simulink model "FOC_CURRENTLOOP_DOUBLE"  (R2024a)
settings: Solver=FixedStepDiscrete  StartTime=0.0  StopTime=10.0  FixedStep=TsBSP  RelTol=1e-3
values from neighbouring files (symbols this model uses):
  bandwidth = 1256.6370614359173    [FOC_CURRENTLOOP_DOUBLE.sldd]
  flux = 0.0109    [FOC_CURRENTLOOP_DOUBLE.sldd]
  Ls = 0.000195185    [FOC_CURRENTLOOP_DOUBLE.sldd]
  Polepairs = 5.0    [FOC_CURRENTLOOP_DOUBLE.sldd]
  Polepairs_MODEL = 5.0    [FOC_CURRENTLOOP_DOUBLE.sldd]
  PWMHalfPeriod = 4199.0    [FOC_CURRENTLOOP_DOUBLE.sldd]
  PWMHalfPeriod_MODEL = 4199.0    [FOC_CURRENTLOOP_DOUBLE.sldd]
  Rs = 0.1763    [FOC_CURRENTLOOP_DOUBLE.sldd]
  TsBSP = 5.0E-5    [FOC_CURRENTLOOP_DOUBLE.sldd]
  TsFOC = 0.0001    [FOC_CURRENTLOOP_DOUBLE.sldd]
undefined symbols (not defined in the file or in its folder): sigbuilder_block
libraries: slpidlib x2, mcbplantlib x1, SignalEditorBlockLib x1, autolibpmsmexterior x1
(part 1 of 2)
settings Model: DataDictionary=FOC_CURRENTLOOP_DOUBLE.sldd  Creator=beau_  LastModifiedBy=chaoli_wanjietian
settings SolverCC: AlgebraicLoopSolver=TrustRegion
settings OptimizationCC: DefaultParameterBehavior=Inlined  UseDivisionForNetSlopeComputation=on  GainParamInheritBuiltInType=on  UseFloatMulNetSlope=on  InlineInvariantSignals=on  PassReuseOutputArgsAs=Individual arguments  ZeroExternalMemoryAtStartup=off  ZeroInternalMemoryAtStartup=off  NoFixptDivByZeroProtection=on  EfficientFloat2IntCast=on  LifeSpan=1  OptimizeBlockOrder=speed  DifferentSizesBufferReuse=on  EfficientTunableParamExpr=on
settings DebuggingCC: ParameterTunabilityLossMsg=error  UnconnectedInputMsg=warning  UnconnectedOutputMsg=warning  UnconnectedLineMsg=warning  BusObjectLabelMismatch=error
settings HardwareCC: ProdBitPerPointer=32  ProdBitPerSizeT=32  ProdBitPerPtrDiffT=32  ProdLargestAtomicInteger=Long  ProdLargestAtomicFloat=Double  ProdWordSize=32  ProdLongLongMode=on  ProdHWDeviceType=ARM Compatible->ARM Cortex-M
settings ModelReferenceCC: EnableRefExpFcnMdlSchedulingChecks=on
settings SFSimCC: SimUserIncludeDirs=E:\Exp_G431\NUM1_CURRENTLOOP\  MATLABDynamicMemAlloc=off
settings SFSimCC: SimCustomHeaderCode=|
  | #include "jscl_transform.h"
  | #include "jscl_currentloop.h"
settings SFSimCC: SimUserSources=|
  | jscl_transform.c
  | jscl_currentloop.c
settings RTWCC: Description=Embedded Coder  SystemTargetFile=ert.tlc  GenCodeOnly=on  TemplateMakefile=ert_default_tmf  GenerateReport=on  CustomInclude=E:\Exp_G431\NUM1_CURRENTLOOP  IncludeHyperlinkInReport=on  LaunchReport=on  GenerateTraceInfo=on  GPUComputeCapability=3.5  DLArmComputeVersion=19.05
settings RTWCC: CustomHeaderCode=|
  | #include "jscl_clarke.h"
  | #include "jscl_park.h"
settings RTWCC: CustomSource=|
  | jscl_clarke.c
  | jscl_park.c
settings CodeAppCC: GenerateComments=off  IgnoreCustomStorageClasses=off  OperatorAnnotations=on  SimulinkDataObjDesc=on  SFDataObjDesc=on  CustomSymbolStrGlobalVar=rt$N$M  CustomSymbolStrType=$N$M  CustomSymbolStrFcn=$N$M$F  CustomSymbolStrFcnArg=param_$I$N$M  CustomSymbolStrBlkIO=local_$N$M  CustomSymbolStrMacro=$N$M  SimulinkBlockComments=off
settings ERTTargetCC: TargetLangStandard=C99 (ISO)  CodeReplacementLibrary=ARM Cortex-M  GenerateSampleERTMain=on  IncludeMdlTerminateFcn=off  CombineSignalStateStructs=on  SuppressErrorStatus=on  SupportNonFinite=off  SupportComplex=off  InlinedParameterPlacement=NonHierarchical  ERTCustomFileTemplate=example_file_process.tlc  EnableDataOwnership=on  ERTFilePackagingFormat=CompactWithDataFile  IndentSize=4

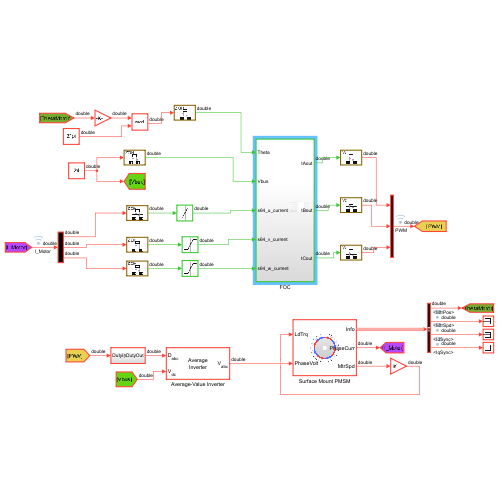
[thumbnail: Simulink's stored preview of the top-level diagram]
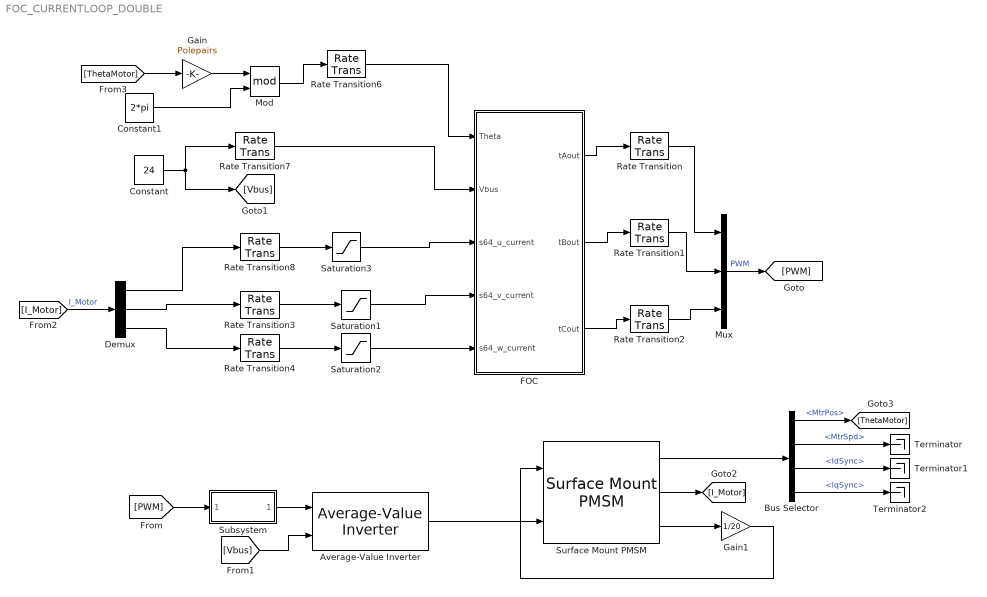
== system FOC_CURRENTLOOP_DOUBLE ==
  Average-Value Inverter : mcbplantlib/Average-Value Inverter
  Bus Selector : BusSelector  OutputSignals=MtrPos,MtrSpd,IdSync,IqSync
  Constant : Constant  Value=24  SampleTime=-1
  Constant1 : Constant  Value=2*pi  SampleTime=-1
  Demux : Demux  Outputs=3
  FOC : Subsystem
  Gain : Gain  Gain=Polepairs
  Gain1 : Gain  Gain=1/20
  Mod : Math  Operator=mod
  Mux : Mux  Inputs=3
  Rate Transition{,1..4,6..8} (8 alike) : RateTransition
  Saturation1 : Saturate  UpperLimit=50  LowerLimit=-50
  Saturation2 : Saturate  UpperLimit=50  LowerLimit=-50
  Saturation3 : Saturate  UpperLimit=50  LowerLimit=-50
  Subsystem : Subsystem
  Surface Mount PMSM : autolibpmsmexterior/Surface Mount PMSM  port_config=Torque  sim_type=Discrete  Ts=TsBSP  P=Polepairs_MODEL  Rs=Rs_MODEL  Ldq_=Ls_MODEL  KConstText=Permanent flux linkage constant (lambda_pm):  lambda_pm=flux_MODEL  Ke=159.9771  Kt=1.323  mechanical=[5.8e-4, 1.59e-4, 0]  idq0=[0 0]  theta_init=0  omega_init=0  KConst=flux_MODEL  lambda_pm_calc=flux_MODEL  RefBlkName='autolibpmsmexterior/Surface Mount PMSM'  aMode=5  Ldq="[0.0017      0.0017]"
  Terminator : Terminator
  Terminator1 : Terminator
  Terminator2 : Terminator
  wires:
  Rate Transition6/1 -> FOC/1(Theta)
  FOC/1(tAout) -> Rate Transition/1
  FOC/2(tBout) -> Rate Transition1/1
  FOC/3(tCout) -> Rate Transition2/1
  Average-Value Inverter/1 -> Surface Mount PMSM/2
  Rate Transition1/1 -> Mux/2
  Rate Transition/1 -> Mux/1
  Rate Transition2/1 -> Mux/3
  Mux/1 -> [PWM]  "PWM"
  [PWM] -> Subsystem/1(DutyIn)
  Subsystem/1(DutyOut) -> Average-Value Inverter/1
  Constant/1 -> [Vbus], Rate Transition7/1
  [Vbus] -> Average-Value Inverter/2
  Surface Mount PMSM/1 -> Bus Selector/1
  Bus Selector/1 -> [ThetaMotor]  "<MtrPos>"
  [ThetaMotor] -> Gain/1
  Gain/1 -> Mod/1
  Mod/1 -> Rate Transition6/1
  Constant1/1 -> Mod/2
  Bus Selector/2 -> Terminator/1  "<MtrSpd>"
  Bus Selector/3 -> Terminator1/1  "<IdSync>"
  Bus Selector/4 -> Terminator2/1  "<IqSync>"
  Surface Mount PMSM/3 -> Gain1/1
  Gain1/1 -> Surface Mount PMSM/1
  Rate Transition7/1 -> FOC/2(Vbus)
  Rate Transition8/1 -> Saturation3/1
  Surface Mount PMSM/2 -> [I_Motor]
  Rate Transition3/1 -> Saturation1/1
  Saturation1/1 -> FOC/4(s64_v_current)
  Saturation2/1 -> FOC/5(s64_w_current)
  Rate Transition4/1 -> Saturation2/1
  Saturation3/1 -> FOC/3(s64_u_current)
  [I_Motor] -> Demux/1  "I_Motor"
  Demux/2 -> Rate Transition3/1
  Demux/3 -> Rate Transition4/1
  Demux/1 -> Rate Transition8/1

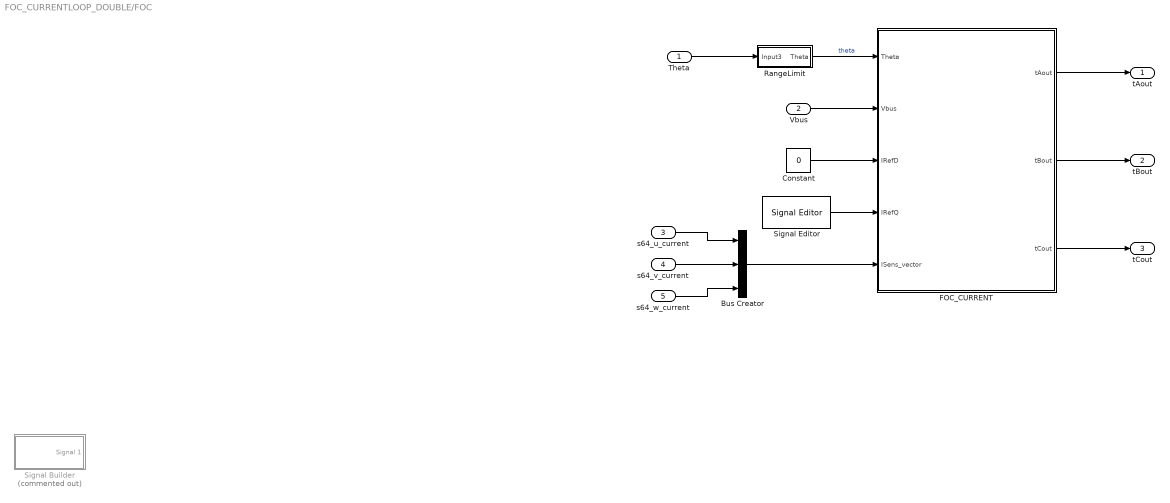
== system FOC_CURRENTLOOP_DOUBLE/FOC ==
  Theta : Inport
  Vbus : Inport  Port=2
  s64_u_current : Inport  Port=3
  s64_v_current : Inport  Port=4
  s64_w_current : Inport  Port=5
  Bus Creator : BusCreator  Inputs=3  OutDataTypeStr=Bus: VectorUVW_T
      settings: InheritFromInputs=off
  Constant : Constant  Value=0  SampleTime=-1
  FOC_CURRENT : Subsystem  TreatAsAtomicUnit=on  SystemSampleTime=TsFOC
      settings: RTWSystemCode=Nonreusable function
  RangeLimit : Subsystem
  Signal Builder : Subsystem  Tag=STV Subsys  Commented=on  LoadFcn=sigbuilder_block('load');  StartFcn=sigbuilder_block('start');  StopFcn=sigbuilder_block('stop');  ClipboardFcn=sigbuilder_block('clipboard');  mask(Sigbuilder block){tuvar=[0:10]}
      mask help: Simulink:masks:SigbuilderBlock_MD
      mask init:
      | if ~strcmp(get_param(bdroot(gcbh),'SimulationStatus'),'stopped') tuvar = sigbuilder_block('maskInit'); end
      settings: CopyFcn=sigbuilder_block('copy');  DeleteFcn=sigbuilder_block('delete');  ModelCloseFcn=sigbuilder_block('modelClose');  PreSaveFcn=sigbuilder_block('preSave');  PauseFcn=sigbuilder_block('pause');  ContinueFcn=sigbuilder_block('continue');  NameChangeFcn=sigbuilder_block('namechange');  OpenFcn=sigbuilder_block('open',[261 231.5 550.5 362.5 ]);  CloseFcn=sigbuilder_block('close');
      mask Display: plot(0, 0, 100, 100,[2, 2, 32, 32, 2], [68, 8, 8, 68, 68],[32, 2], [38, 38], [32, 19, 2],[53, 60, 44], [32, 17, 17, 2],[16, 16, 31, 31]);txt = getActiveGroup(gcbh);text(2, 100, txt,'verticalAlignment', 'top');
  Signal Editor : SignalEditorBlockLib/Signal Editor  FileName=E:\Exp_G431\NUM1_CURRENTLOOP\builder_edit.mat  ActiveScenario=Scenario  ActiveSignal=IRefQ  IsBus=off  OutputBusObjectStr=Bus: BusObject  SampleTime=TsFOC  Interpolate=off  ZeroCross=off  OutputAfterFinalValue=Setting to zero  Unit=inherit  PreserveSignalName=on  ApplySigPropsToAllScenarios=on  ApplySigPropsToAllSignals=off
  tAout : Outport
  tBout : Outport  Port=2
  tCout : Outport  Port=3
  wires:
  Vbus/1 -> FOC_CURRENT/2(Vbus)
  Theta/1 -> RangeLimit/1(Input3)
  RangeLimit/1(Theta) -> FOC_CURRENT/1(Theta)  "theta"
  Constant/1 -> FOC_CURRENT/3(IRefD)
  Signal Editor/1 -> FOC_CURRENT/4(IRefQ)
  Bus Creator/1 -> FOC_CURRENT/5(ISens_vector)
  s64_u_current/1 -> Bus Creator/1
  s64_v_current/1 -> Bus Creator/2
  s64_w_current/1 -> Bus Creator/3
  FOC_CURRENT/3(tCout) -> tCout/1
  FOC_CURRENT/2(tBout) -> tBout/1
  FOC_CURRENT/1(tAout) -> tAout/1

== system FOC_CURRENTLOOP_DOUBLE/Subsystem ==
  DutyIn : Inport
  Constant : Constant  Value=0.5
  Gain : Gain  Gain=1/PWMHalfPeriod_MODEL
  Gain1 : Gain  Gain=-1
  Sum : Sum  Inputs=|+-
  Sum1 : Sum  Inputs=|++
  DutyOut : Outport
  wires:
  DutyIn/1 -> Gain/1
  Gain/1 -> Sum/1
  Sum/1 -> Gain1/1
  Gain1/1 -> Sum1/1
  Sum1/1 -> DutyOut/1
  Constant/1 -> Sum1/2, Sum/2

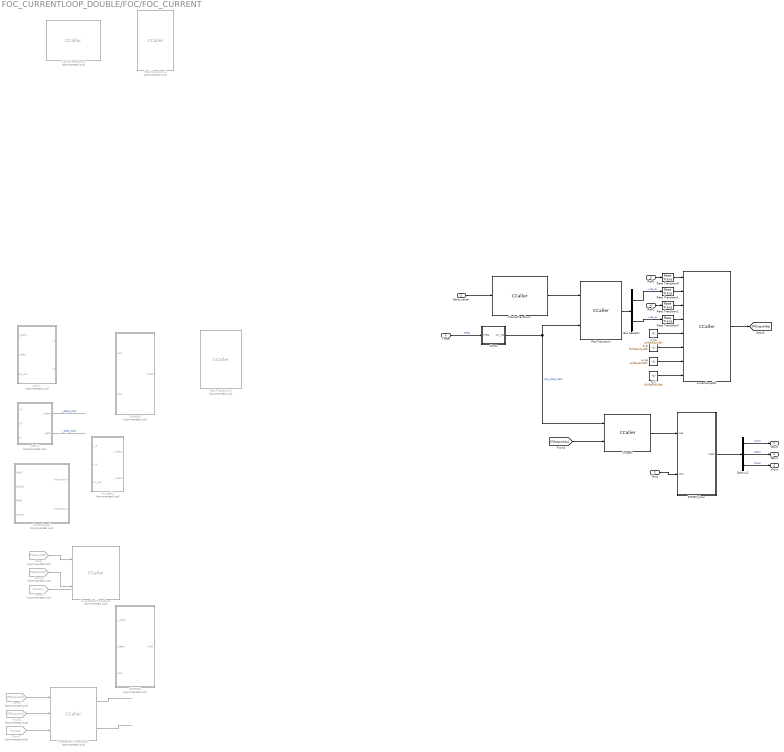
== system FOC_CURRENTLOOP_DOUBLE/FOC/FOC_CURRENT ==
  Theta : Inport
  Vbus : Inport  Port=2
  IRefD : Inport  Port=3
  IRefQ : Inport  Port=4
  ISens_vector : Inport  Port=5  OutDataTypeStr=Bus: VectorUVW_T
  Bus Selector : BusSelector  OutputSignals=s64_d,s64_q
  ClarkeTransform : CCaller  FunctionName=ClarkeTransform  PortSpecificationStruct="%)30     .    Z ,   8    (     @         %    \"     (    !     0         %  0 \"0    $    _    07)G3F%M90  4&]R=$YA;64 4V-O<&4     26YD97@     5'EP90      4VEZ90      27-';&]B86P   X    X    !@    @    $          4    (     0    8    !         !     &    04)#7VEN   .    .     8    (    !          %    \"     $    &     0         0    !@   $%\"0U]I;@  #@   #@    &    \"     0         !0    @    !    !0    $         $     4   !);G!U=     X    X    !@    @    &          4    (     0    $    !          D    (               .    0     8    (    !          %    \"     $    0     0         0    $    $)U<SH@5F5C=&]R55977U0.    ,     8    (    !          %    \"     $    !     0         0  $ ,0    X    P    !@    @    ) @        4    (     0    $    !          (  0      #@   #@    &    \"     0         !0    @    !    !@    $         $     8   !!0E]O=70   X    X    !@    @    $          4    (     0    8    !         !     &    04)?;W5T   .    .     8    (    !          %    \"     $    &     0         0    !@   $]U='!U=   #@   #@    &    \"     8         !0    @    !     0    $         \"0    @               X   !     !@    @    $          4    (     0    \\    !         !     /    0G5S.B!696-T;W)!0E]4  X    P    !@    @    $          4    (     0    $    !         !   0 Q    #@   #     &    \"     D\"        !0    @    !     0    $          @ !"
  ClarkeTransform1 : CCaller  Commented=on  FunctionName=ClarkeTransform  PortSpecificationStruct="%)30     .    H 4   8    (     @         %    \"     ,    !     0         %  0 \"0    $    _    07)G3F%M90  4&]R=$YA;64 4V-O<&4     26YD97@     5'EP90      4VEZ90      27-';&]B86P   X   !     !@    @    $          4    (     0    D    !         !     )    :6Y?=F5C=&]R          X   !     !@    @    $          4    (     0    D    !         !     )    :6Y?=F5C=&]R          X    X    !@    @    $          4    (     0    4    !         !     %    26YP=70    .    .     8    (    !@         %    \"     $    !     0         )    \"               #@   $     &    \"     0         !0    @    !    $     $         $    !    !\"=7,Z($-L87)K94EN<'5T#@   #     &    \"     0         !0    @    !     0    $         $  ! #$    .    ,     8    (    \"0(        %    \"     $    !     0         \"  $       X    X    !@    @    $          4    (     0    <    !         !     '    :5]A;'!H80 .    .     8    (    !          %    \"     $    '     0         0    !P   &E?86QP:&$ #@   #@    &    \"     0         !0    @    !    !@    $         $     8   !/=71P=70   X    X    !@    @    &          4    (     0    $    !          D    (               .    .     8    (    !          %    \"     $    &     0         0    !@   &1O=6)L90  #@   #     &    \"     0         !0    @    !     0    $         $  ! #$    .    ,     8    (    \"0(        %    \"     $    !     0         \"  $       X    X    !@    @    $          4    (     0    8    !         !     &    :5]B971A   .    .     8    (    !          %    \"     $    &     0         0    !@   &E?8F5T80  #@   #@    &    \"     0         !0    @    !    !@    $         $     8   !/=71P=70   X    X    !@    @    &          4    (     0    $    !          D    (            \\#\\.    .     8    (    !          %    \"     $    &     0         0    !@   &1O=6)L90  #@   #     &    \"     0         !0    @    !     0    $         $  ! #$    .    ,     8    (    \"0(        %    \"     $    !     0         \"  $"
  CurrentLoop1 : Subsystem  Commented=on  TreatAsAtomicUnit=on
      settings: RTWSystemCode=Nonreusable function
  Demux2 : Demux  Outputs=3
  From : From  Commented=on  GotoTag=PIOutputVd
  From1 : From  Commented=on  GotoTag=PIOutputVq
  From2 : From  Commented=on  GotoTag=sincos
  From5 : From  Commented=on  GotoTag=PIOutputVd
  From6 : From  Commented=on  GotoTag=PIOutputVq
  From7 : From  Commented=on  GotoTag=sincos
  InverseParkTransform : CCaller  Commented=on  FunctionName=InverseParkTransform  PortSpecificationStruct="%)30     .    F 4   8    (     @         %    \"     ,    !     0         %  0 \"0    $    _    07)G3F%M90  4&]R=$YA;64 4V-O<&4     26YD97@     5'EP90      4VEZ90      27-';&]B86P   X    X    !@    @    $          4    (     0    4    !         !     %    1%%?:6X    .    .     8    (    !          %    \"     $    %     0         0    !0   $117VEN    #@   #@    &    \"     0         !0    @    !    !0    $         $     4   !);G!U=     X    X    !@    @    &          4    (     0    $    !          D    (               .    0     8    (    !          %    \"     $    /     0         0    #P   $)U<SH@5F5C=&]R1%%?5  .    ,     8    (    !          %    \"     $    !     0         0  $ ,0    X    P    !@    @    ) @        4    (     0    $    !          (  0      #@   #@    &    \"     0         !0    @    !    !0    $         $     4   !T:&5T80    X    X    !@    @    $          4    (     0    4    !         !     %    =&AE=&$    .    .     8    (    !          %    \"     $    %     0         0    !0   $EN<'5T    #@   #@    &    \"     8         !0    @    !     0    $         \"0    @           #P/PX    X    !@    @    $          4    (     0    8    !         !     &    9&]U8FQE   .    ,     8    (    !          %    \"     $    !     0         0  $ ,0    X    P    !@    @    ) @        4    (     0    $    !          (  0      #@   #@    &    \"     0         !0    @    !    !@    $         $     8   !!0E]O=70   X    X    !@    @    $          4    (     0    8    !         !     &    04)?;W5T   .    .     8    (    !          %    \"     $    &     0         0    !@   $]U='!U=   #@   #@    &    \"     8         !0    @    !     0    $         \"0    @               X   !     !@    @    $          4    (     0    \\    !         !     /    0G5S.B!696-T;W)!0E]4  X    P    !@    @    $          4    (     0    $    !         !   0 Q    #@   #     &    \"     D\"        !0    @    !     0    $          @ !"
  InverseParkTransform1 : CCaller  Commented=on  FunctionName=InverseParkTransform  PortSpecificationStruct="%)30     .    T @   8    (     @         %    \"     4    !     0         %  0 \"0    $    _    07)G3F%M90  4&]R=$YA;64 4V-O<&4     26YD97@     5'EP90      4VEZ90      27-';&]B86P   X    P    !@    @    $          4    (     0    ,    !         !   P!U7V0 #@   #     &    \"     0         !0    @    !     P    $         $  # '5?9  .    .     8    (    !          %    \"     $    %     0         0   ...(+2661 chars)"
  ParkTransform : CCaller  FunctionName=ParkTransform  PortSpecificationStruct="%)30     .    F 4   8    (     @         %    \"     ,    !     0         %  0 \"0    $    _    07)G3F%M90  4&]R=$YA;64 4V-O<&4     26YD97@     5'EP90      4VEZ90      27-';&]B86P   X    X    !@    @    $          4    (     0    4    !         !     %    04)?:6X    .    .     8    (    !          %    \"     $    %     0         0    !0   $%\"7VEN    #@   #@    &    \"     0         !0    @    !    !0    $         $     4   !);G!U=     X    X    !@    @    &          4    (     0    $    !          D    (               .    0     8    (    !          %    \"     $    /     0         0    #P   $)U<SH@5F5C=&]R04)?5  .    ,     8    (    !          %    \"     $    !     0         0  $ ,0    X    P    !@    @    ) @        4    (     0    $    !          (  0      #@   #@    &    \"     0         !0    @    !    !P    $         $     <   !S:6Y?8V]S  X    X    !@    @    $          4    (     0    <    !         !     '    <VEN7V-O<P .    .     8    (    !          %    \"     $    %     0         0    !0   $EN<'5T    #@   #@    &    \"     8         !0    @    !     0    $         \"0    @           #P/PX    X    !@    @    $          4    (     0    8    !         !     &    9&]U8FQE   .    ,     8    (    !          %    \"     $    !     0         0  $ ,@    X    P    !@    @    ) @        4    (     0    $    !          (  0      #@   #@    &    \"     0         !0    @    !    !@    $         $     8   !$45]O=70   X    X    !@    @    $          4    (     0    8    !         !     &    1%%?;W5T   .    .     8    (    !          %    \"     $    &     0         0    !@   $]U='!U=   #@   #@    &    \"     8         !0    @    !     0    $         \"0    @               X   !     !@    @    $          4    (     0    \\    !         !     /    0G5S.B!696-T;W)$45]4  X    P    !@    @    $          4    (     0    $    !         !   0 Q    #@   #     &    \"     D\"        !0    @    !     0    $          @ !"
  ParkTransform1 : CCaller  Commented=on  FunctionName=ParkTransform  PortSpecificationStruct="%)30     .    T @   8    (     @         %    \"     4    !     0         %  0 \"0    $    _    07)G3F%M90  4&]R=$YA;64 4V-O<&4     26YD97@     5'EP90      4VEZ90      27-';&]B86P   X    X    !@    @    $          4    (     0    <    !         !     '    :5]A;'!H80 .    .     8    (    !          %    \"     $    '     0         0    !P   &E?86QP:&$ #@   #@    &    \"     0         !0    @    !   ...(+2659 chars)"
  ParkTransform2 : CCaller  Commented=on  FunctionName=ParkTransform  PortSpecificationStruct="%)30     .    F 4   8    (     @         %    \"     ,    !     0         %  0 \"0    $    _    07)G3F%M90  4&]R=$YA;64 4V-O<&4     26YD97@     5'EP90      4VEZ90      27-';&]B86P   X    X    !@    @    $          4    (     0    4    !         !     %    04)?:6X    .    .     8    (    !          %    \"     $    %     0         0    !0   $%\"7VEN    #@   #@    &    \"     0         !0    @    !    !0    $         $     4   !);G!U=     X    X    !@    @    &          4    (     0    $    !          D    (               .    0     8    (    !          %    \"     $    /     0         0    #P   $)U<SH@5F5C=&]R04)?5  .    ,     8    (    !          %    \"     $    !     0         0  $ ,0    X    P    !@    @    ) @        4    (     0    $    !          (  0      #@   #@    &    \"     0         !0    @    !    !0    $         $     4   !T:&5T80    X    X    !@    @    $          4    (     0    4    !         !     %    =&AE=&$    .    .     8    (    !          %    \"     $    %     0         0    !0   $EN<'5T    #@   #@    &    \"     8         !0    @    !     0    $         \"0    @           #P/PX    X    !@    @    $          4    (     0    8    !         !     &    9&]U8FQE   .    ,     8    (    !          %    \"     $    !     0         0  $ ,0    X    P    !@    @    ) @        4    (     0    $    !          (  0      #@   #@    &    \"     0         !0    @    !    !@    $         $     8   !$45]O=70   X    X    !@    @    $          4    (     0    8    !         !     &    1%%?;W5T   .    .     8    (    !          %    \"     $    &     0         0    !@   $]U='!U=   #@   #@    &    \"     8         !0    @    !     0    $         \"0    @               X   !     !@    @    $          4    (     0    \\    !         !     /    0G5S.B!696-T;W)$45]4  X    P    !@    @    $          4    (     0    $    !         !   0 Q    #@   #     &    \"     D\"        !0    @    !     0    $          @ !"
  Rate Transition{1..3,8} (4 alike) : RateTransition
  SVPWM2 : Subsystem  Commented=on  TreatAsAtomicUnit=on
      settings: RTWSystemCode=Nonreusable function
  SVPWM3 : Subsystem  Commented=on  TreatAsAtomicUnit=on
  SVPWM_func : Subsystem  TreatAsAtomicUnit=on
      settings: RTWSystemCode=Nonreusable function
  clark1 : Subsystem  Commented=on  TreatAsAtomicUnit=on
      mask Display:
      | port_label('input',1,'a','texmode','on');
      | port_label('input',2,'b','texmode','on');
      | port_label('input',3,'c','texmode','on');
      | 
      | port_label('output',1,'\alpha','texmode','on');
      | port_label('output',2,'\beta','texmode','on');
      | 
      | fprintf('Clark');
  currentLoopDQ : CCaller  FunctionName=CurrentLoopDQ  PortSpecificationStruct="%)30     .    \\ \\   8    (     @         %    \"     D    !     0         %  0 \"0    $    _    07)G3F%M90  4&]R=$YA;64 4V-O<&4     26YD97@     5'EP90      4VEZ90      27-';&]B86P   X    X    !@    @    $          4    (     0    4    !         !     %    25)E9D0    .    .     8    (    !          %    \"     $    %     0         0    !0   $E2969$    #@   #@    &    \"     0         !0    @    ! ...(+5127 chars)"
  d_ki : Constant  Value=Rs*bandwidth  SampleTime=TsFOC
  d_kp : Constant  Value=Ls*bandwidth  SampleTime=TsFOC
  inv_park1 : Subsystem  Commented=on  TreatAsAtomicUnit=on
      settings: RTWSystemCode=Nonreusable function
  invpark : CCaller  FunctionName=InverseParkTransform  PortSpecificationStruct="%)30     .    > 4   8    (     @         %    \"     ,    !     0         %  0 \"0    $    _    07)G3F%M90  4&]R=$YA;64 4V-O<&4     26YD97@     5'EP90      4VEZ90      27-';&]B86P   X    X    !@    @    $          4    (     0    <    !         !     '    <VEN7V-O<P .    .     8    (    !          %    \"     $    '     0         0    !P   '-I;E]C;W, #@   #@    &    \"     0         !0    @    !    !0    $         $     4   !);G!U=     X    X    !@    @    &          4    (     0    $    !          D    (               .    .     8    (    !          %    \"     $    &     0         0    !@   &1O=6)L90  #@   #     &    \"     0         !0    @    !     0    $         $  ! #(    .    ,     8    (    \"0(        %    \"     $    !     0         \"  $       X    P    !@    @    $          4    (     0    (    !         !   @!I;@  #@   #     &    \"     0         !0    @    !     @    $         $  \" &EN   .    .     8    (    !          %    \"     $    %     0         0    !0   $EN<'5T    #@   #@    &    \"     8         !0    @    !     0    $         \"0    @           #P/PX   !     !@    @    $          4    (     0    \\    !         !     /    0G5S.B!696-T;W)$45]4  X    P    !@    @    $          4    (     0    $    !         !   0 Q    #@   #     &    \"     D\"        !0    @    !     0    $          @ !       .    ,     8    (    !          %    \"     $    #     0         0  , ;W5T  X    P    !@    @    $          4    (     0    ,    !         !   P!O=70 #@   #@    &    \"     0         !0    @    !    !@    $         $     8   !/=71P=70   X    X    !@    @    &          4    (     0    $    !          D    (               .    0     8    (    !          %    \"     $    /     0         0    #P   $)U<SH@5F5C=&]R04)?5  .    ,     8    (    !          %    \"     $    !     0         0  $ ,0    X    P    !@    @    ) @        4    (     0    $    !          (  0"
  park1 : Subsystem  Commented=on  TreatAsAtomicUnit=on
  q_ki : Constant  Value=Rs*bandwidth  SampleTime=TsFOC
  q_kp : Constant  Value=Ls*bandwidth  SampleTime=TsFOC
  sincos : Subsystem
  tAout : Outport
  tBout : Outport  Port=2
  tCout : Outport  Port=3
  wires:
  Theta/1 -> sincos/1(theta)  "theta"
  IRefD/1 -> Rate Transition8/1
  IRefQ/1 -> Rate Transition2/1
  From/1 -> InverseParkTransform/1
  Rate Transition8/1 -> currentLoopDQ/1
  clark1/2(i_beta) -> ?  "i_beta_clark"
  clark1/1(i_alpha) -> ?  "i_alpha_clark"
  ? -> clark1/3(i_c)
  ? -> clark1/2(i_b)
  ? -> clark1/1(i_a)
  Rate Transition1/1 -> currentLoopDQ/2
  Rate Transition2/1 -> currentLoopDQ/3
  Rate Transition3/1 -> currentLoopDQ/4
  d_kp/1 -> currentLoopDQ/5
  d_ki/1 -> currentLoopDQ/6
  q_kp/1 -> currentLoopDQ/7
  q_ki/1 -> currentLoopDQ/8
  From1/1 -> InverseParkTransform/2
  From2/1 -> ?
  ParkTransform/1 -> Bus Selector/1
  Bus Selector/1 -> Rate Transition1/1  "<s64_d>"
  Bus Selector/2 -> Rate Transition3/1  "<s64_q>"
  From5/1 -> InverseParkTransform1/1
  InverseParkTransform1/1 -> ?
  From6/1 -> InverseParkTransform1/2
  From7/1 -> InverseParkTransform1/3
  InverseParkTransform1/2 -> ?
  invpark/1 -> SVPWM_func/1(Uαβ)
  Vbus/1 -> SVPWM_func/2(vbus)
  SVPWM_func/1(tABC) -> Demux2/1
  Demux2/2 -> tBout/1  "tBout"
  Demux2/3 -> tCout/1  "tCout"
  Demux2/1 -> tAout/1  "tAout"
  ISens_vector/1 -> ClarkeTransform/1
  ClarkeTransform/1 -> ParkTransform/1
  sincos/1(sin_cos) -> ParkTransform/2, invpark/1  "sine_cose_theta"
  currentLoopDQ/1 -> [PIOutputVdq]
  [PIOutputVdq] -> invpark/2

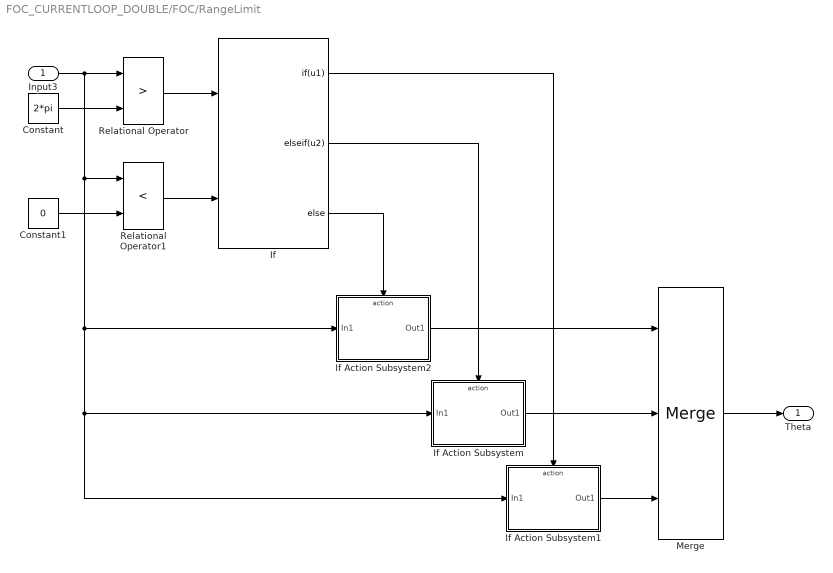
== system FOC_CURRENTLOOP_DOUBLE/FOC/RangeLimit ==
  Input3 : Inport
  Constant : Constant  Value=2*pi  OutDataTypeStr=double  SampleTime=-1
  Constant1 : Constant  Value=0  OutDataTypeStr=double  SampleTime=-1
  If : If  NumInputs=2  IfExpression=u1  ElseIfExpressions=u2
  If Action Subsystem : Subsystem  TreatAsAtomicUnit=on
  If Action Subsystem1 : Subsystem  TreatAsAtomicUnit=on
  If Action Subsystem2 : Subsystem  TreatAsAtomicUnit=on
  Merge : Merge  Inputs=3
  Relational Operator : RelationalOperator  Operator=>  OutDataTypeStr=boolean  RndMeth=Simplest  InputSameDT=off
  Relational Operator1 : RelationalOperator  Operator=<  OutDataTypeStr=boolean  RndMeth=Simplest  InputSameDT=off
  Theta : Outport
  wires:
  Relational Operator/1 -> If/1
  Constant/1 -> Relational Operator/2
  Constant1/1 -> Relational Operator1/2
  Input3/1 -> Relational Operator1/1, If Action Subsystem2/1(In1), If Action Subsystem1/1(In1), If Action Subsystem/1(In1), Relational Operator/1
  Relational Operator1/1 -> If/2
  Merge/1 -> Theta/1
  If/3 -> If Action Subsystem2/Action
  If/2 -> If Action Subsystem/Action
  If/1 -> If Action Subsystem1/Action
  If Action Subsystem2/1(Out1) -> Merge/1
  If Action Subsystem/1(Out1) -> Merge/2
  If Action Subsystem1/1(Out1) -> Merge/3

== system FOC_CURRENTLOOP_DOUBLE/FOC/Signal Builder ==
  Demux : Demux  Tag=STV Demux  Outputs=1
      settings: DisplayOption=none
  FromWs : FromWorkspace  Tag=STV FromWs  VariableName=tuvar
      SigBuilderData=|
      | common.afterFinalStr = 'Extrapolate'
      | common.sampleTime = 0
      | dataSet.timeRange = [0 10]
      | dataSet.name = 'Group 1'
      | sbobj.Groups.Name = 'Group 1'
      | sbobj.Groups.Signals.Name = 'Signal 1'
      | sbobj.Groups.Signals.XData = [0 1.98 1.98 4 4 6 6 10]
      | sbobj.Groups.Signals.YData = [20 20 -20 -20 6.6 6.6 -5.8 -5.8]
  Signal 1 : Outport  Tag=STV Outport
  wires:
  Demux/1 -> Signal 1/1
  FromWs/1 -> Demux/1

== system FOC_CURRENTLOOP_DOUBLE/FOC/FOC_CURRENT/CurrentLoop1 ==
  IRefD : Inport
  ISensD : Inport  Port=2
  IRefQ : Inport  Port=3
  ISensQ : Inport  Port=4
  DCurrentPI : Subsystem  TreatAsAtomicUnit=on
      settings: RTWSystemCode=Nonreusable function
  QCurrentPI : Subsystem  TreatAsAtomicUnit=on
      settings: RTWSystemCode=Nonreusable function
  PIOutoutVd : Outport
  PIOutputVq : Outport  Port=2
  wires:
  IRefD/1 -> DCurrentPI/1(In1)
  ISensD/1 -> DCurrentPI/2(In2)
  DCurrentPI/1(Out1) -> PIOutoutVd/1
  IRefQ/1 -> QCurrentPI/1(In1)
  ISensQ/1 -> QCurrentPI/2(In2)
  QCurrentPI/1(Out1) -> PIOutputVq/1

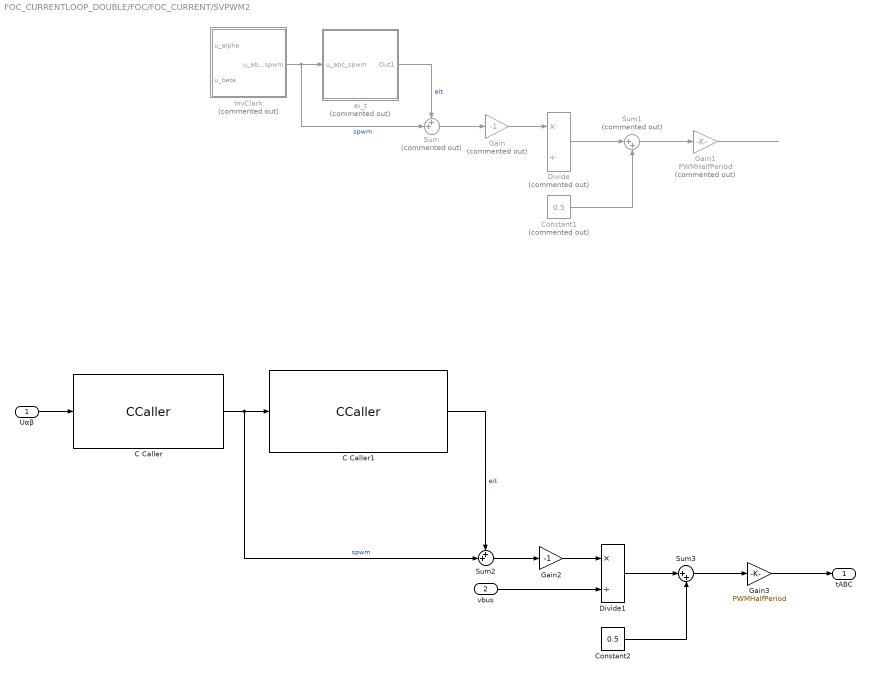
== system FOC_CURRENTLOOP_DOUBLE/FOC/FOC_CURRENT/SVPWM2 ==
  Uαβ : Inport
  vbus : Inport  Port=2
  C Caller : CCaller  FunctionName=InverseClarkeTransform  PortSpecificationStruct="%)30     .    Z ,   8    (     @         %    \"     (    !     0         %  0 \"0    $    _    07)G3F%M90  4&]R=$YA;64 4V-O<&4     26YD97@     5'EP90      4VEZ90      27-';&]B86P   X    X    !@    @    $          4    (     0    4    !         !     %    04)?:6X    .    .     8    (    !          %    \"     $    %     0         0    !0   $%\"7VEN    #@   #@    &    \"     0         !0    @    !    !0    $         $     4   !);G!U=     X    X    !@    @    &          4    (     0    $    !          D    (               .    0     8    (    !          %    \"     $    /     0         0    #P   $)U<SH@5F5C=&]R04)?5  .    ,     8    (    !          %    \"     $    \"     0         0  ( +3$   X    P    !@    @    ) @        4    (     0    $    !          (  0      #@   #@    &    \"     0         !0    @    !    !P    $         $     <   !!0D-?;W5T  X    X    !@    @    $          4    (     0    <    !         !     '    04)#7V]U=  .    .     8    (    !          %    \"     $    &     0         0    !@   $]U='!U=   #@   #@    &    \"     8         !0    @    !     0    $         \"0    @               X   !     !@    @    $          4    (     0   !     !         !     0    0G5S.B!696-T;W)55E=?5 X    P    !@    @    $          4    (     0    $    !         !   0 Q    #@   #     &    \"     D\"        !0    @    !     0    $          @ !"
  C Caller1 : CCaller  FunctionName=CalcZeroSequenceVoltage  PortSpecificationStruct="%)30     .    X ,   8    (     @         %    \"     (    !     0         %  0 \"0    $    _    07)G3F%M90  4&]R=$YA;64 4V-O<&4     26YD97@     5'EP90      4VEZ90      27-';&]B86P   X    X    !@    @    $          4    (     0    4    !         !     %    =5]A8F,    .    .     8    (    !          %    \"     $    %     0         0    !0   '5?86)C    #@   #@    &    \"     0         !0    @    !    !0    $         $     4   !);G!U=     X    X    !@    @    &          4    (     0    $    !          D    (               .    0     8    (    !          %    \"     $    0     0         0    $    $)U<SH@5F5C=&]R55977U0.    ,     8    (    !          %    \"     $    !     0         0  $ ,0    X    P    !@    @    ) @        4    (     0    $    !          (  0      #@   #@    &    \"     0         !0    @    !    !@    $         $     8   !U7WIE<F\\   X    X    !@    @    $          4    (     0    8    !         !     &    =5]Z97)O   .    .     8    (    !          %    \"     $    &     0         0    !@   $]U='!U=   #@   #@    &    \"     8         !0    @    !     0    $         \"0    @               X    X    !@    @    $          4    (     0    8    !         !     &    9&]U8FQE   .    ,     8    (    !          %    \"     $    !     0         0  $ ,0    X    P    !@    @    ) @        4    (     0    $    !          (  0"
  Constant1 : Constant  Commented=on  Value=0.5  SampleTime=TsFOC
  Constant2 : Constant  Value=0.5  SampleTime=TsFOC
  Divide : Product  Commented=on  Inputs=*/
  Divide1 : Product  Inputs=*/
  Gain : Gain  Commented=on  Gain=-1
  Gain1 : Gain  Commented=on  Gain=PWMHalfPeriod
  Gain2 : Gain  Gain=-1
  Gain3 : Gain  Gain=PWMHalfPeriod
  InvClark : Subsystem  Commented=on  TreatAsAtomicUnit=on
      settings: RTWSystemCode=Nonreusable function
  Sum : Sum  Commented=on  Inputs=++|
  Sum1 : Sum  Commented=on  Inputs=|++
  Sum2 : Sum  Inputs=++|
  Sum3 : Sum  Inputs=|++
  ei_t : Subsystem  Commented=on  TreatAsAtomicUnit=on
      settings: RTWSystemCode=Nonreusable function
  tABC : Outport
  wires:
  ei_t/1(Out1) -> Sum/1  "eit"
  InvClark/1(u_abc_spwm) -> Sum/2, ei_t/1(u_abc_spwm)  "spwm"
  Sum/1 -> Gain/1
  Gain/1 -> Divide/1
  Divide/1 -> Sum1/1
  Constant1/1 -> Sum1/2
  Sum1/1 -> Gain1/1
  Gain1/1 -> ?
  Gain3/1 -> tABC/1
  Constant2/1 -> Sum3/2
  Sum3/1 -> Gain3/1
  Gain2/1 -> Divide1/1
  Sum2/1 -> Gain2/1
  vbus/1 -> Divide1/2
  Divide1/1 -> Sum3/1
  C Caller/1 -> Sum2/2, C Caller1/1  "spwm"
  C Caller1/1 -> Sum2/1  "eit"
  Uαβ/1 -> C Caller/1

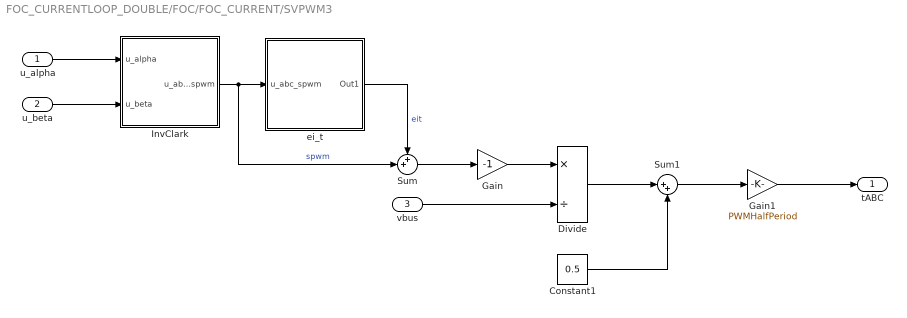
== system FOC_CURRENTLOOP_DOUBLE/FOC/FOC_CURRENT/SVPWM3 ==
  u_alpha : Inport
  u_beta : Inport  Port=2
  vbus : Inport  Port=3
  Constant1 : Constant  Value=0.5  OutDataTypeStr=single  SampleTime=-1
  Divide : Product  Inputs=*/
  Gain : Gain  Gain=-1
  Gain1 : Gain  Gain=PWMHalfPeriod
  InvClark : Subsystem
  Sum : Sum  Inputs=++|
  Sum1 : Sum  Inputs=|++
  ei_t : Subsystem
  tABC : Outport
  wires:
  u_alpha/1 -> InvClark/1(u_alpha)
  u_beta/1 -> InvClark/2(u_beta)
  ei_t/1(Out1) -> Sum/1  "eit"
  InvClark/1(u_abc_spwm) -> Sum/2, ei_t/1(u_abc_spwm)  "spwm"
  Sum/1 -> Gain/1
  Gain/1 -> Divide/1
  vbus/1 -> Divide/2
  Divide/1 -> Sum1/1
  Constant1/1 -> Sum1/2
  Sum1/1 -> Gain1/1
  Gain1/1 -> tABC/1

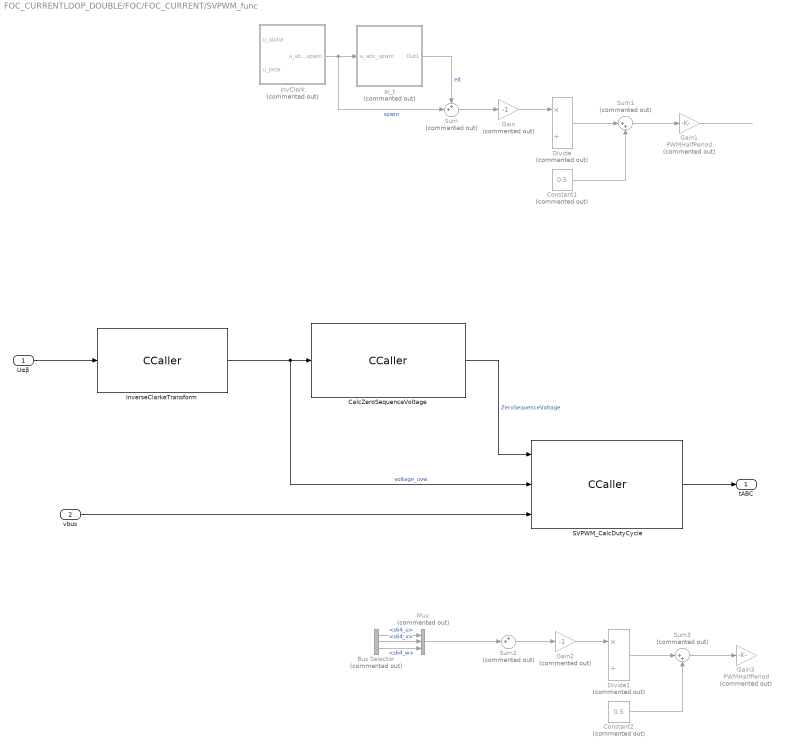
== system FOC_CURRENTLOOP_DOUBLE/FOC/FOC_CURRENT/SVPWM_func ==
  Uαβ : Inport
  vbus : Inport  Port=2
  Bus Selector : BusSelector  Commented=on  OutputSignals=s64_u,s64_v,s64_w
  CalcZeroSequenceVoltage : CCaller  FunctionName=CalcZeroSequenceVoltage  PortSpecificationStruct="%)30     .    X ,   8    (     @         %    \"     (    !     0         %  0 \"0    $    _    07)G3F%M90  4&]R=$YA;64 4V-O<&4     26YD97@     5'EP90      4VEZ90      27-';&]B86P   X    X    !@    @    $          4    (     0    4    !         !     %    =5]A8F,    .    .     8    (    !          %    \"     $    %     0         0    !0   '5?86)C    #@   #@    &    \"     0         !0    @    !    !0    $         $     4   !);G!U=     X    X    !@    @    &          4    (     0    $    !          D    (               .    0     8    (    !          %    \"     $    0     0         0    $    $)U<SH@5F5C=&]R55977U0.    ,     8    (    !          %    \"     $    !     0         0  $ ,0    X    P    !@    @    ) @        4    (     0    $    !          (  0      #@   #@    &    \"     0         !0    @    !    !@    $         $     8   !U7WIE<F\\   X    X    !@    @    $          4    (     0    8    !         !     &    =5]Z97)O   .    .     8    (    !          %    \"     $    &     0         0    !@   $]U='!U=   #@   #@    &    \"     8         !0    @    !     0    $         \"0    @               X    X    !@    @    $          4    (     0    8    !         !     &    9&]U8FQE   .    ,     8    (    !          %    \"     $    !     0         0  $ ,0    X    P    !@    @    ) @        4    (     0    $    !          (  0"
  Constant1 : Constant  Commented=on  Value=0.5  SampleTime=TsFOC
  Constant2 : Constant  Commented=on  Value=0.5  OutDataTypeStr=single  SampleTime=-1
  Divide : Product  Commented=on  Inputs=*/
  Divide1 : Product  Commented=on  Inputs=*/
  Gain : Gain  Commented=on  Gain=-1
  Gain1 : Gain  Commented=on  Gain=PWMHalfPeriod
  Gain2 : Gain  Commented=on  Gain=-1
  Gain3 : Gain  Commented=on  Gain=PWMHalfPeriod
  InvClark : Subsystem  Commented=on  TreatAsAtomicUnit=on
      settings: RTWSystemCode=Nonreusable function
  InverseClarkeTransform : CCaller  FunctionName=InverseClarkeTransform  PortSpecificationStruct="%)30     .    Z ,   8    (     @         %    \"     (    !     0         %  0 \"0    $    _    07)G3F%M90  4&]R=$YA;64 4V-O<&4     26YD97@     5'EP90      4VEZ90      27-';&]B86P   X    X    !@    @    $          4    (     0    4    !         !     %    04)?:6X    .    .     8    (    !          %    \"     $    %     0         0    !0   $%\"7VEN    #@   #@    &    \"     0         !0    @    !    !0    $         $     4   !);G!U=     X    X    !@    @    &          4    (     0    $    !          D    (               .    0     8    (    !          %    \"     $    /     0         0    #P   $)U<SH@5F5C=&]R04)?5  .    ,     8    (    !          %    \"     $    !     0         0  $ ,0    X    P    !@    @    ) @        4    (     0    $    !          (  0      #@   #@    &    \"     0         !0    @    !    !P    $         $     <   !!0D-?;W5T  X    X    !@    @    $          4    (     0    <    !         !     '    04)#7V]U=  .    .     8    (    !          %    \"     $    &     0         0    !@   $]U='!U=   #@   #@    &    \"     8         !0    @    !     0    $         \"0    @               X   !     !@    @    $          4    (     0   !     !         !     0    0G5S.B!696-T;W)55E=?5 X    P    !@    @    $          4    (     0    $    !         !   0 Q    #@   #     &    \"     D\"        !0    @    !     0    $          @ !"
  Mux : Mux  Commented=on  Inputs=3
  SVPWM_CalcDutyCycle : CCaller  FunctionName=SVPWM_CalcDutyCycle  PortSpecificationStruct="%)30     .    ( <   8    (     @         %    \"     0    !     0         %  0 \"0    $    _    07)G3F%M90  4&]R=$YA;64 4V-O<&4     26YD97@     5'EP90      4VEZ90      27-';&]B86P   X    X    !@    @    $          4    (     0    8    !         !     &    =5]Z97)O   .    .     8    (    !          %    \"     $    &     0         0    !@   '5?>F5R;P  #@   #@    &    \"     0         !0    @    !   ...(+2075 chars)"
  Sum : Sum  Commented=on  Inputs=++|
  Sum1 : Sum  Commented=on  Inputs=|++
  Sum2 : Sum  Commented=on  Inputs=++|
  Sum3 : Sum  Commented=on  Inputs=|++
  ei_t : Subsystem  Commented=on  TreatAsAtomicUnit=on
      settings: RTWSystemCode=Nonreusable function
  tABC : Outport
  wires:
  ei_t/1(Out1) -> Sum/1  "eit"
  InvClark/1(u_abc_spwm) -> Sum/2, ei_t/1(u_abc_spwm)  "spwm"
  Sum/1 -> Gain/1
  Gain/1 -> Divide/1
  Divide/1 -> Sum1/1
  Constant1/1 -> Sum1/2
  Sum1/1 -> Gain1/1
  Gain1/1 -> ?
  InverseClarkeTransform/1 -> SVPWM_CalcDutyCycle/2, CalcZeroSequenceVoltage/1  "voltage_uvw"
  Uαβ/1 -> InverseClarkeTransform/1
  Sum3/1 -> Gain3/1
  Sum2/1 -> Gain2/1
  Gain2/1 -> Divide1/1
  Divide1/1 -> Sum3/1
  Constant2/1 -> Sum3/2
  Mux/1 -> Sum2/2
  Bus Selector/1 -> Mux/1  "<s64_u>"
  Bus Selector/2 -> Mux/2  "<s64_v>"
  Bus Selector/3 -> Mux/3  "<s64_w>"
  vbus/1 -> SVPWM_CalcDutyCycle/3
  CalcZeroSequenceVoltage/1 -> SVPWM_CalcDutyCycle/1  "ZeroSequenceVoltage"
  SVPWM_CalcDutyCycle/1 -> tABC/1
